simulink model "TriTiltPro_V3"  (R2019a)
settings: Solver=ode15s  StartTime=0.0  StopTime=1  RelTol=1e-3  EnableMultiTasking=on
undefined symbols (not defined in the file or in its folder): magnitude, sigbuilder_block, X, Y, Z
libraries: sm_lib x405, nesl_utility x28, simulink x13, fl_lib x7, fl_ps_legacy_lib x6, sharedtransform x1, Multibody_Multiphysics_Lib x1
(part 1 of 9)
settings Model: Creator=Administrator  LastModifiedBy=SomefunAgba
settings SolverCC: InitialStep=0.001  ZeroCrossControl=EnableAll  ZeroCrossAlgorithm=Adaptive  InsertRTBMode=Never (minimum delay)
settings DataIOCC: LimitDataPoints=on  SaveFinalState=on  SaveFormat=StructureWithTime  SaveState=on  SignalLogging=off  InspectSignalLogs=on  OutputOption=SpecifiedOutputTimes  OutputTimes=[0:1/30:1]
settings OptimizationCC: BlockReduction=off  BufferReuse=off  LifeSpan=1  MaxStackSize=64
settings DebuggingCC: SFUnexpectedBacktrackingDiag=warning  SFNoUnconditionalDefaultTransitionDiag=warning  ArithmeticOperatorsInVariantConditions=warning
settings HardwareCC: ProdBitPerPointer=32  ProdBitPerSizeT=32  ProdBitPerPtrDiffT=32  ProdLargestAtomicFloat=None  ProdIntDivRoundTo=Undefined  ProdEndianess=Unspecified  ProdWordSize=32  ProdHWDeviceType=Generic->Unspecified (assume 32-bit Generic)  TargetHWDeviceType=32-bit Generic
settings ModelReferenceCC: PropagateSignalLabelsOutOfModel=off
settings SFSimCC: SimUseLocalCustomCode=off  MATLABDynamicMemAlloc=off
settings RTWCC: SystemTargetFile=ert.tlc  HardwareBoard=Robot Operating System (ROS)  TLCOptions=-aInlineSetEventsForThisBaseRateFcn=TLC_FALSE -aSuppressMultiTaskScheduler=TLC_FALSE -aRateBasedStepFcn=0  TemplateMakefile=ert_default_tmf  GenerateReport=on  RTWUseLocalCustomCode=off  Toolchain=Catkin  IncludeHyperlinkInReport=on  LaunchReport=on  TargetLang=C++  GenerateTraceInfo=on  GenerateTraceReport=on  GenerateTraceReportSl=on  GenerateTraceReportSf=on  GenerateTraceReportEml=on
settings CodeAppCC: ForceParamTrailComments=on  IgnoreCustomStorageClasses=off  OperatorAnnotations=on  SimulinkDataObjDesc=on  SFDataObjDesc=on  MATLABFcnDesc=on  InsertBlockDesc=on  StateflowObjectComments=on  MATLABSourceComments=on
settings ERTTargetCC: MultiwordLength=2048
settings ConfigComp: CovMetricSettings=dw  CovHtmlReporting=on  CovSaveCumulativeToWorkspaceVar=on  CovSaveSingleToWorkspaceVar=on  CovExternalEMLEnable=off
settings SimscapeCC: SimscapeNormalizeSystem=off  SimscapeLogType=all  SimscapeLogSimulationStatistics=on  SimscapeLogOpenViewer=on
settings SimMechanicsCC: VisDuringSimulation=on
settings ConfigurationSet: Description=SimMechanics 2G
settings ExplorerConfigSet: InternalSimMechanicsExplorerSettings="<ExplorerConfiguration><canonicalview>planar_xy</canonicalview><AnimationSetting><BasePlaybackSpeed>1.0</BasePlaybackSpeed><PlaybackSpeedFactor>1.0</PlaybackSpeedFactor></AnimationSetting><TilePanel><TileInfo><Tiles Columns=\"1\" Count=\"1\" Rows=\"1\"><Column Left=\"2\" Weight=\"1\"/><Column Left=\"705\"/><Row Top=\"2\" Weight=\"1\"/><Row Top=\"457\"/><Tile Height=\"1\" Width=\"1\" X=\"0\" Y=\"0\"/></Tiles></TileInfo><SceneInfo><SceneViewer><BGColor><R>0.60000002384185791</R><G>0.80000001192092896</G><B>1</B></BGColor><Camera><Position><X>369622.51927765959</X><Y>14452.522627350738</Y><Z>-4093.5800779968113</Z></Position><Center><X>-0.26213935017585754</X><Y>0.48995256423950195</Y><Z>-0.58916831016540527</Z></Center><Up><X>-0.039071238740294556</X><Y>0.99923641605206415</Y><Z>-0.00015211418458100246</Z></Up><Left>-1.18166543841362</Left><Right>1.18166543841362</Right><Bottom>-0.63869556784629822</Bottom><Top>0.63869556784629822</Top></Camera></SceneViewer></SceneInfo></TilePanel></ExplorerConfiguration>"

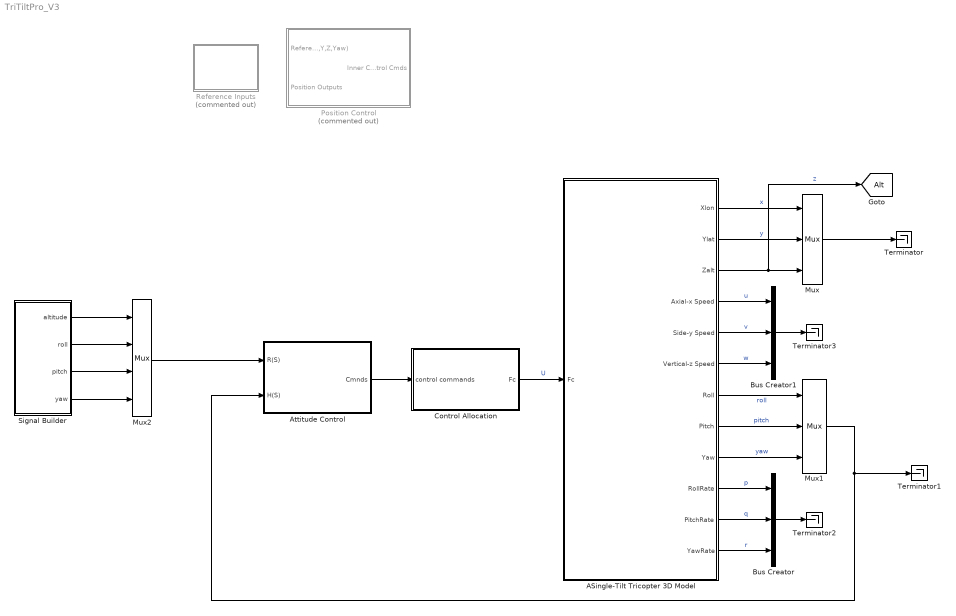
== system TriTiltPro_V3 ==
  ASingle-Tilt Tricopter 3D Model : Subsystem
  Attitude Control : Subsystem
  Bus Creator : BusCreator  Inputs=3
  Bus Creator1 : BusCreator  Inputs=3
  Control Allocation : Subsystem
  Mux : Mux  Inputs=3
  Mux1 : Mux  Inputs=3
  Mux2 : Mux
  Position Control : Subsystem  Commented=on
  Reference Inputs : Subsystem  Commented=on
  Signal Builder : Subsystem  Tag=STV Subsys  LoadFcn=sigbuilder_block('load');  StartFcn=sigbuilder_block('start');  StopFcn=sigbuilder_block('stop');  ClipboardFcn=sigbuilder_block('clipboard');  mask(Sigbuilder block){tuvar=[0:10]}
      mask help: Simulink:masks:SigbuilderBlock_MD
      mask init:
      | if ~strcmp(get_param(bdroot(gcbh),'SimulationStatus'),'stopped') tuvar = sigbuilder_block('maskInit'); end
      settings: CopyFcn=sigbuilder_block('copy');  DeleteFcn=sigbuilder_block('delete');  ModelCloseFcn=sigbuilder_block('modelClose');  PreSaveFcn=sigbuilder_block('preSave');  PauseFcn=sigbuilder_block('pause');  ContinueFcn=sigbuilder_block('continue');  NameChangeFcn=sigbuilder_block('namechange');  OpenFcn=sigbuilder_block('open',[299.25 91.5 558 358.5 ]);  CloseFcn=sigbuilder_block('close');
      mask Display: plot(0, 0, 100, 100,[2, 2, 32, 32, 2], [68, 8, 8, 68, 68],[32, 2], [38, 38], [32, 19, 2],[53, 60, 44], [32, 17, 17, 2],[16, 16, 31, 31]);txt = getActiveGroup(gcbh);text(2, 100, txt,'verticalAlignment', 'top');
  Terminator{,1..3} (4 alike) : Terminator
  tag scope: Alt=global
  wires:
  ASingle-Tilt Tricopter 3D Model/12(YawRate) -> Bus Creator/3  "r"
  ASingle-Tilt Tricopter 3D Model/11(PitchRate) -> Bus Creator/2  "q"
  ASingle-Tilt Tricopter 3D Model/10(RollRate) -> Bus Creator/1  "p"
  ASingle-Tilt Tricopter 3D Model/9(Yaw) -> Mux1/3  "yaw"
  ASingle-Tilt Tricopter 3D Model/8(Pitch) -> Mux1/2  "pitch"
  ASingle-Tilt Tricopter 3D Model/7(Roll) -> Mux1/1  "roll"
  ASingle-Tilt Tricopter 3D Model/6(Vertical-z Speed) -> Bus Creator1/3  "w"
  ASingle-Tilt Tricopter 3D Model/5(Side-y Speed) -> Bus Creator1/2  "v"
  ASingle-Tilt Tricopter 3D Model/4(Axial-x Speed) -> Bus Creator1/1  "u"
  ASingle-Tilt Tricopter 3D Model/3(Zalt) -> [Alt], Mux/3  "z"
  ASingle-Tilt Tricopter 3D Model/2(Ylat) -> Mux/2  "y"
  ASingle-Tilt Tricopter 3D Model/1(Xlon) -> Mux/1  "x"
  Mux/1 -> Terminator/1
  Mux1/1 -> Attitude Control/2(H(S)), Terminator1/1
  Control Allocation/1(Fc) -> ASingle-Tilt Tricopter 3D Model/1(Fc)  "U"
  Attitude Control/1(Cmnds) -> Control Allocation/1(control commands)
  Mux2/1 -> Attitude Control/1(R(S))
  Signal Builder/1(altitude) -> Mux2/1
  Signal Builder/2(roll) -> Mux2/2
  Signal Builder/3(pitch) -> Mux2/3
  Signal Builder/4(yaw) -> Mux2/4
  Bus Creator/1 -> Terminator2/1
  Bus Creator1/1 -> Terminator3/1

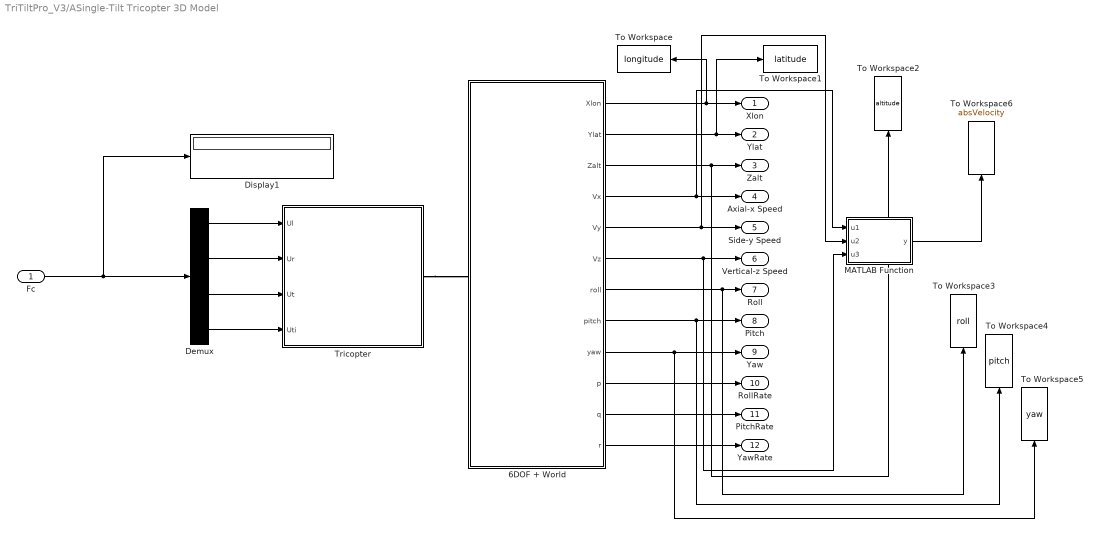
== system TriTiltPro_V3/ASingle-Tilt Tricopter 3D Model ==
  Fc : Inport
  6DOF + World : Subsystem
  Demux : Demux
  Display1 : Display
  MATLAB Function : MATLAB Function  TreatAsAtomicUnit=on
  To Workspace : ToWorkspace  VariableName=longitude  SampleTime=-1
  To Workspace1 : ToWorkspace  VariableName=latitude  SampleTime=-1
  To Workspace2 : ToWorkspace  VariableName=altitude  SampleTime=-1
  To Workspace3 : ToWorkspace  VariableName=roll  SampleTime=-1
  To Workspace4 : ToWorkspace  VariableName=pitch  SampleTime=-1
  To Workspace5 : ToWorkspace  VariableName=yaw  SampleTime=-1
  To Workspace6 : ToWorkspace  VariableName=absVelocity  SampleTime=-1
  Tricopter : Subsystem
  Xlon : Outport
  Ylat : Outport  Port=2
  Zalt : Outport  Port=3
  Axial-x Speed : Outport  Port=4
  Side-y Speed : Outport  Port=5
  Vertical-z Speed : Outport  Port=6
  Roll : Outport  Port=7
  Pitch : Outport  Port=8
  Yaw : Outport  Port=9
  RollRate : Outport  Port=10
  PitchRate : Outport  Port=11
  YawRate : Outport  Port=12
  wires:
  6DOF + World/9(yaw) -> To Workspace5/1, Yaw/1
  6DOF + World/10(p) -> RollRate/1
  6DOF + World/4(Vx) -> MATLAB Function/1(u1), Axial-x Speed/1
  6DOF + World/3(Zalt) -> To Workspace2/1, Zalt/1
  6DOF + World/11(q) -> PitchRate/1
  6DOF + World/12(r) -> YawRate/1
  6DOF + World/6(Vz) -> MATLAB Function/3(u3), Vertical-z Speed/1
  6DOF + World/2(Ylat) -> To Workspace1/1, Ylat/1
  6DOF + World/7(roll) -> To Workspace3/1, Roll/1
  6DOF + World/8(pitch) -> To Workspace4/1, Pitch/1
  6DOF + World/5(Vy) -> MATLAB Function/2(u2), Side-y Speed/1
  6DOF + World/1(Xlon) -> To Workspace/1, Xlon/1
  Demux/3 -> Tricopter/3(Ut)
  Demux/1 -> Tricopter/1(Ul)
  Demux/4 -> Tricopter/4(Uti)
  Demux/2 -> Tricopter/2(Ur)
  Fc/1 -> Display1/1, Demux/1
  MATLAB Function/1(y) -> To Workspace6/1
  connections:
  Tricopter/RConn1 -- 6DOF + World/LConn1

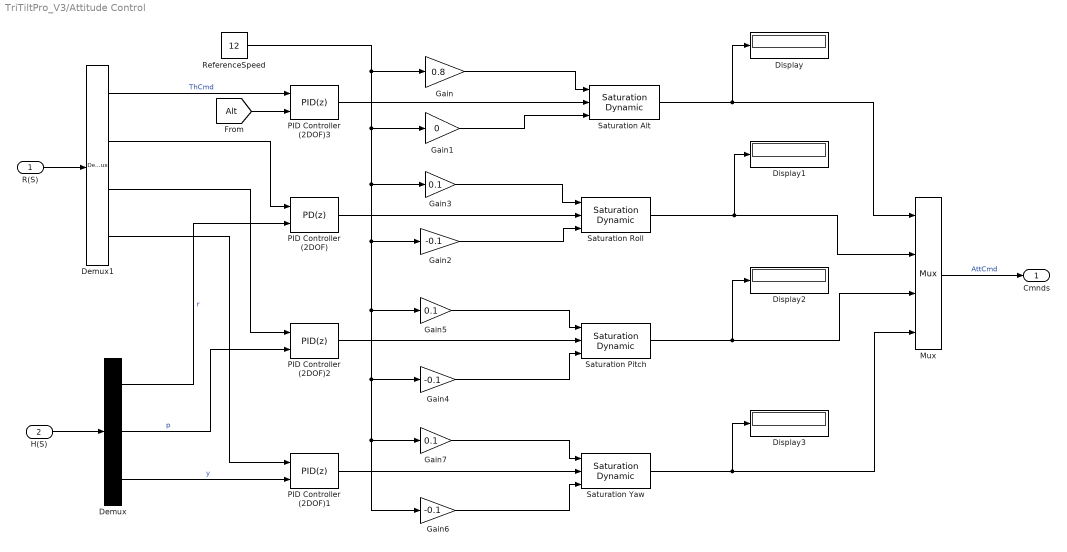
== system TriTiltPro_V3/Attitude Control ==
  R(S) : Inport
  H(S) : Inport  Port=2
  Demux : Demux  Outputs=3
  Demux1 : Demux
  Display{,1..3} (4 alike) : Display
  Gain : Gain  Gain=0.8
  Gain1 : Gain  Gain=0
  Gain2 : Gain  Gain=-0.1
  Gain3 : Gain  Gain=0.1
  Gain4 : Gain  Gain=-0.1
  Gain5 : Gain  Gain=0.1
  Gain6 : Gain  Gain=-0.1
  Gain7 : Gain  Gain=0.1
  Mux : Mux
  PID Controller (2DOF) : simulink/Continuous/PID Controller (2DOF)  Controller=PD  Form=Parallel  TimeDomain=Discrete-time  SampleTime=0.001  IntegratorMethod=Forward Euler  FilterMethod=Forward Euler  ControllerParametersSource=internal  P=21.0891711051547  I=1  D=0  UseFilter=on  N=100  b=0  c=1  TunerSelectOption=Transfer Function Based (PID Tuner App)  InitialConditionSource=internal  InitialConditionForIntegrator=0  InitialConditionForFilter=0  DifferentiatorICPrevScaledInput=0  ExternalReset=none  TrackingMode=off  Kt=1  LimitOutput=off  UpperSaturationLimit=inf  LowerSaturationLimit=-inf  LinearizeAsGain=on  AntiWindupMode=none  Kb=1  POutMin=[]  POutMax=[]  IOutMin=[]  IOutMax=[]  DOutMin=[]  DOutMax=[]  NOutMin=[]  NOutMax=[]  bOutMin=[]  bOutMax=[]  cOutMin=[]  cOutMax=[]  SumOutMin=[]  SumOutMax=[]  SaturationOutMin=[]  SaturationOutMax=[]  PParamMin=[]  PParamMax=[]  IParamMin=[]  IParamMax=[]  DParamMin=[]  DParamMax=[]  NParamMin=[]  NParamMax=[]  bParamMin=[]  bParamMax=[]  cParamMin=[]  cParamMax=[]  KbParamMin=[]  KbParamMax=[]  KtParamMin=[]  KtParamMax=[]  KbOutMin=[]  KbOutMax=[]  KtOutMin=[]  KtOutMax=[]  IntegratorOutMin=[]  IntegratorOutMax=[]  FilterOutMin=[]  FilterOutMax=[]  SumI1OutMin=[]  SumI1OutMax=[]  SumI2OutMin=[]  SumI2OutMax=[]  SumI3OutMin=[]  SumI3OutMax=[]  SumI4OutMin=[]  SumI4OutMax=[]  SumDOutMin=[]  SumDOutMax=[]  Sum1OutMin=[]  Sum1OutMax=[]  Sum2OutMin=[]  Sum2OutMax=[]  Sum3OutMin=[]  Sum3OutMax=[]  DifferentiatorOutMin=[]  DifferentiatorOutMax=[]  FilterDiffOutCoefMin=[]  FilterDiffOutCoefMax=[]  ReciprocalOutMin=[]  ReciprocalOutMax=[]  SumDenOutMin=[]  SumDenOutMax=[]  SumNumOutMin=[]  SumNumOutMax=[]  DivideOutMin=[]  DivideOutMax=[]  IntegratorContinuousStateAttributes=''  IntegratorStateMustResolveToSignalObject=off  IntegratorRTWStateStorageClass=Auto  FilterContinuousStateAttributes=''  FilterStateMustResolveToSignalObject=off  FilterRTWStateStorageClass=Auto  ParallelPVariant=InternalParameters  IdealPVariant=Disabled  IVariant=Disabled  DVariant=InternalParameters  bVariant=InternalParameters  cVariant=InternalParameters  IntegratorVariant=Disabled  SatVariant=Disabled  AWVariant=Disabled  PCopyVariant=Disabled  TRVariant=Disabled  FdbkBlocksVariant=Forward  IdealPFdbkVariant=Disabled  SatFdbkVariant=Disabled  DerivativeFilterVariant=ForwardEulerFilter  NVariant=InternalParameters  NCopyVariant=Disabled  FilterICVariant=InternalICsFilter  IntegratorICVariant=Disabled  ExternalResetVariant=Disabled  TRSumVariant=Passthrough  SumFdbkVariant=Disabled  SumVariant=Sum_PD
  PID Controller (2DOF)1 : simulink/Continuous/PID Controller (2DOF)  Controller=PID  Form=Parallel  TimeDomain=Discrete-time  SampleTime=0.001  IntegratorMethod=Forward Euler  FilterMethod=Forward Euler  ControllerParametersSource=internal  P=0.02  I=0.4  D=0.001  UseFilter=on  N=1730.43460231117  b=0.949409560304364  c=0.478998391491009  TunerSelectOption=Transfer Function Based (PID Tuner App)  InitialConditionSource=internal  InitialConditionForIntegrator=0  InitialConditionForFilter=0  DifferentiatorICPrevScaledInput=0  ExternalReset=none  TrackingMode=off  Kt=1  LimitOutput=off  UpperSaturationLimit=inf  LowerSaturationLimit=-inf  LinearizeAsGain=on  AntiWindupMode=none  Kb=1  POutMin=[]  POutMax=[]  IOutMin=[]  IOutMax=[]  DOutMin=[]  DOutMax=[]  NOutMin=[]  NOutMax=[]  bOutMin=[]  bOutMax=[]  cOutMin=[]  cOutMax=[]  SumOutMin=[]  SumOutMax=[]  SaturationOutMin=[]  SaturationOutMax=[]  PParamMin=[]  PParamMax=[]  IParamMin=[]  IParamMax=[]  DParamMin=[]  DParamMax=[]  NParamMin=[]  NParamMax=[]  bParamMin=[]  bParamMax=[]  cParamMin=[]  cParamMax=[]  KbParamMin=[]  KbParamMax=[]  KtParamMin=[]  KtParamMax=[]  KbOutMin=[]  KbOutMax=[]  KtOutMin=[]  KtOutMax=[]  IntegratorOutMin=[]  IntegratorOutMax=[]  FilterOutMin=[]  FilterOutMax=[]  SumI1OutMin=[]  SumI1OutMax=[]  SumI2OutMin=[]  SumI2OutMax=[]  SumI3OutMin=[]  SumI3OutMax=[]  SumI4OutMin=[]  SumI4OutMax=[]  SumDOutMin=[]  SumDOutMax=[]  Sum1OutMin=[]  Sum1OutMax=[]  Sum2OutMin=[]  Sum2OutMax=[]  Sum3OutMin=[]  Sum3OutMax=[]  DifferentiatorOutMin=[]  DifferentiatorOutMax=[]  FilterDiffOutCoefMin=[]  FilterDiffOutCoefMax=[]  ReciprocalOutMin=[]  ReciprocalOutMax=[]  SumDenOutMin=[]  SumDenOutMax=[]  SumNumOutMin=[]  SumNumOutMax=[]  DivideOutMin=[]  DivideOutMax=[]  IntegratorContinuousStateAttributes=''  IntegratorStateMustResolveToSignalObject=off  IntegratorRTWStateStorageClass=Auto  FilterContinuousStateAttributes=''  FilterStateMustResolveToSignalObject=off  FilterRTWStateStorageClass=Auto  ParallelPVariant=InternalParameters  IdealPVariant=Disabled  IVariant=InternalParameters  DVariant=InternalParameters  bVariant=InternalParameters  cVariant=InternalParameters  IntegratorVariant=Discrete  SatVariant=Disabled  AWVariant=Passthrough  PCopyVariant=Disabled  TRVariant=Disabled  FdbkBlocksVariant=Forward  IdealPFdbkVariant=Disabled  SatFdbkVariant=Disabled  DerivativeFilterVariant=ForwardEulerFilter  NVariant=InternalParameters  NCopyVariant=Disabled  FilterICVariant=InternalICsFilter  IntegratorICVariant=InternalICs  ExternalResetVariant=Disabled  TRSumVariant=Passthrough  SumFdbkVariant=Disabled  SumVariant=Sum_PID
  PID Controller (2DOF)2 : simulink/Continuous/PID Controller (2DOF)  Controller=PID  Form=Parallel  TimeDomain=Discrete-time  SampleTime=0.001  IntegratorMethod=Forward Euler  FilterMethod=Forward Euler  ControllerParametersSource=internal  P=0.02  I=0.4  D=0.001  UseFilter=on  N=100  b=1  c=1  TunerSelectOption=Transfer Function Based (PID Tuner App)  InitialConditionSource=internal  InitialConditionForIntegrator=0  InitialConditionForFilter=0  DifferentiatorICPrevScaledInput=0  ExternalReset=none  TrackingMode=off  Kt=1  LimitOutput=off  UpperSaturationLimit=inf  LowerSaturationLimit=-inf  LinearizeAsGain=on  AntiWindupMode=none  Kb=1  POutMin=[]  POutMax=[]  IOutMin=[]  IOutMax=[]  DOutMin=[]  DOutMax=[]  NOutMin=[]  NOutMax=[]  bOutMin=[]  bOutMax=[]  cOutMin=[]  cOutMax=[]  SumOutMin=[]  SumOutMax=[]  SaturationOutMin=[]  SaturationOutMax=[]  PParamMin=[]  PParamMax=[]  IParamMin=[]  IParamMax=[]  DParamMin=[]  DParamMax=[]  NParamMin=[]  NParamMax=[]  bParamMin=[]  bParamMax=[]  cParamMin=[]  cParamMax=[]  KbParamMin=[]  KbParamMax=[]  KtParamMin=[]  KtParamMax=[]  KbOutMin=[]  KbOutMax=[]  KtOutMin=[]  KtOutMax=[]  IntegratorOutMin=[]  IntegratorOutMax=[]  FilterOutMin=[]  FilterOutMax=[]  SumI1OutMin=[]  SumI1OutMax=[]  SumI2OutMin=[]  SumI2OutMax=[]  SumI3OutMin=[]  SumI3OutMax=[]  SumI4OutMin=[]  SumI4OutMax=[]  SumDOutMin=[]  SumDOutMax=[]  Sum1OutMin=[]  Sum1OutMax=[]  Sum2OutMin=[]  Sum2OutMax=[]  Sum3OutMin=[]  Sum3OutMax=[]  DifferentiatorOutMin=[]  DifferentiatorOutMax=[]  FilterDiffOutCoefMin=[]  FilterDiffOutCoefMax=[]  ReciprocalOutMin=[]  ReciprocalOutMax=[]  SumDenOutMin=[]  SumDenOutMax=[]  SumNumOutMin=[]  SumNumOutMax=[]  DivideOutMin=[]  DivideOutMax=[]  IntegratorContinuousStateAttributes=''  IntegratorStateMustResolveToSignalObject=off  IntegratorRTWStateStorageClass=Auto  FilterContinuousStateAttributes=''  FilterStateMustResolveToSignalObject=off  FilterRTWStateStorageClass=Auto  ParallelPVariant=InternalParameters  IdealPVariant=Disabled  IVariant=InternalParameters  DVariant=InternalParameters  bVariant=InternalParameters  cVariant=InternalParameters  IntegratorVariant=Discrete  SatVariant=Disabled  AWVariant=Passthrough  PCopyVariant=Disabled  TRVariant=Disabled  FdbkBlocksVariant=Forward  IdealPFdbkVariant=Disabled  SatFdbkVariant=Disabled  DerivativeFilterVariant=ForwardEulerFilter  NVariant=InternalParameters  NCopyVariant=Disabled  FilterICVariant=InternalICsFilter  IntegratorICVariant=InternalICs  ExternalResetVariant=Disabled  TRSumVariant=Passthrough  SumFdbkVariant=Disabled  SumVariant=Sum_PID
  PID Controller (2DOF)3 : simulink/Continuous/PID Controller (2DOF)  Controller=PID  Form=Parallel  TimeDomain=Discrete-time  SampleTime=0.001  IntegratorMethod=Forward Euler  FilterMethod=Forward Euler  ControllerParametersSource=internal  P=15.9810269634034  I=1121.61470890408  D=0  UseFilter=on  N=100  b=1  c=1  TunerSelectOption=Transfer Function Based (PID Tuner App)  InitialConditionSource=internal  InitialConditionForIntegrator=0  InitialConditionForFilter=0  DifferentiatorICPrevScaledInput=0  ExternalReset=none  TrackingMode=off  Kt=1  LimitOutput=off  UpperSaturationLimit=inf  LowerSaturationLimit=-inf  LinearizeAsGain=on  AntiWindupMode=none  Kb=1  POutMin=[]  POutMax=[]  IOutMin=[]  IOutMax=[]  DOutMin=[]  DOutMax=[]  NOutMin=[]  NOutMax=[]  bOutMin=[]  bOutMax=[]  cOutMin=[]  cOutMax=[]  SumOutMin=[]  SumOutMax=[]  SaturationOutMin=[]  SaturationOutMax=[]  PParamMin=[]  PParamMax=[]  IParamMin=[]  IParamMax=[]  DParamMin=[]  DParamMax=[]  NParamMin=[]  NParamMax=[]  bParamMin=[]  bParamMax=[]  cParamMin=[]  cParamMax=[]  KbParamMin=[]  KbParamMax=[]  KtParamMin=[]  KtParamMax=[]  KbOutMin=[]  KbOutMax=[]  KtOutMin=[]  KtOutMax=[]  IntegratorOutMin=[]  IntegratorOutMax=[]  FilterOutMin=[]  FilterOutMax=[]  SumI1OutMin=[]  SumI1OutMax=[]  SumI2OutMin=[]  SumI2OutMax=[]  SumI3OutMin=[]  SumI3OutMax=[]  SumI4OutMin=[]  SumI4OutMax=[]  SumDOutMin=[]  SumDOutMax=[]  Sum1OutMin=[]  Sum1OutMax=[]  Sum2OutMin=[]  Sum2OutMax=[]  Sum3OutMin=[]  Sum3OutMax=[]  DifferentiatorOutMin=[]  DifferentiatorOutMax=[]  FilterDiffOutCoefMin=[]  FilterDiffOutCoefMax=[]  ReciprocalOutMin=[]  ReciprocalOutMax=[]  SumDenOutMin=[]  SumDenOutMax=[]  SumNumOutMin=[]  SumNumOutMax=[]  DivideOutMin=[]  DivideOutMax=[]  IntegratorContinuousStateAttributes=''  IntegratorStateMustResolveToSignalObject=off  IntegratorRTWStateStorageClass=Auto  FilterContinuousStateAttributes=''  FilterStateMustResolveToSignalObject=off  FilterRTWStateStorageClass=Auto  ParallelPVariant=InternalParameters  IdealPVariant=Disabled  IVariant=InternalParameters  DVariant=InternalParameters  bVariant=InternalParameters  cVariant=InternalParameters  IntegratorVariant=Discrete  SatVariant=Disabled  AWVariant=Passthrough  PCopyVariant=Disabled  TRVariant=Disabled  FdbkBlocksVariant=Forward  IdealPFdbkVariant=Disabled  SatFdbkVariant=Disabled  DerivativeFilterVariant=ForwardEulerFilter  NVariant=InternalParameters  NCopyVariant=Disabled  FilterICVariant=InternalICsFilter  IntegratorICVariant=InternalICs  ExternalResetVariant=Disabled  TRSumVariant=Passthrough  SumFdbkVariant=Disabled  SumVariant=Sum_PID
  ReferenceSpeed : Constant  Value=12
  Saturation Alt : simulink/Discontinuities/Saturation Dynamic  OutMin=[]  OutMax=[]  OutDataTypeStr=Inherit: Same as second input  OutDataType=fixdt(1, 16)  OutScaling=2^-10  DoSatur=off
  Saturation Pitch : simulink/Discontinuities/Saturation Dynamic  OutMin=[]  OutMax=[]  OutDataTypeStr=Inherit: Same as second input  OutDataType=fixdt(1, 16)  OutScaling=2^-10  DoSatur=off
  Saturation Roll : simulink/Discontinuities/Saturation Dynamic  OutMin=[]  OutMax=[]  OutDataTypeStr=Inherit: Same as second input  OutDataType=fixdt(1, 16)  OutScaling=2^-10  DoSatur=off
  Saturation Yaw : simulink/Discontinuities/Saturation Dynamic  OutMin=[]  OutMax=[]  OutDataTypeStr=Inherit: Same as second input  OutDataType=fixdt(1, 16)  OutScaling=2^-10  DoSatur=off
  Cmnds : Outport
  wires:
  H(S)/1 -> Demux/1
  R(S)/1 -> Demux1/1
  Gain/1 -> Saturation Alt/1
  Gain1/1 -> Saturation Alt/3
  PID Controller (2DOF)3/1 -> Saturation Alt/2
  PID Controller (2DOF)/1 -> Saturation Roll/2
  Gain3/1 -> Saturation Roll/1
  Gain2/1 -> Saturation Roll/3
  PID Controller (2DOF)2/1 -> Saturation Pitch/2
  Gain5/1 -> Saturation Pitch/1
  Gain4/1 -> Saturation Pitch/3
  Mux/1 -> Cmnds/1  "AttCmd"
  Saturation Alt/1 -> Display/1, Mux/1
  Saturation Roll/1 -> Mux/2, Display1/1
  Saturation Pitch/1 -> Mux/3, Display2/1
  ReferenceSpeed/1 -> Gain7/1, Gain6/1, Gain4/1, Gain5/1, Gain2/1, Gain3/1, Gain1/1, Gain/1
  PID Controller (2DOF)1/1 -> Saturation Yaw/2
  Gain7/1 -> Saturation Yaw/1
  Gain6/1 -> Saturation Yaw/3
  Saturation Yaw/1 -> Mux/4, Display3/1
  Demux1/1 -> PID Controller (2DOF)3/1  "ThCmd"
  Demux/3 -> PID Controller (2DOF)1/2  "y"
  Demux1/4 -> PID Controller (2DOF)1/1
  Demux/2 -> PID Controller (2DOF)2/2  "p"
  Demux1/3 -> PID Controller (2DOF)2/1
  Demux/1 -> PID Controller (2DOF)/2  "r"
  Demux1/2 -> PID Controller (2DOF)/1
  [Alt] -> PID Controller (2DOF)3/2

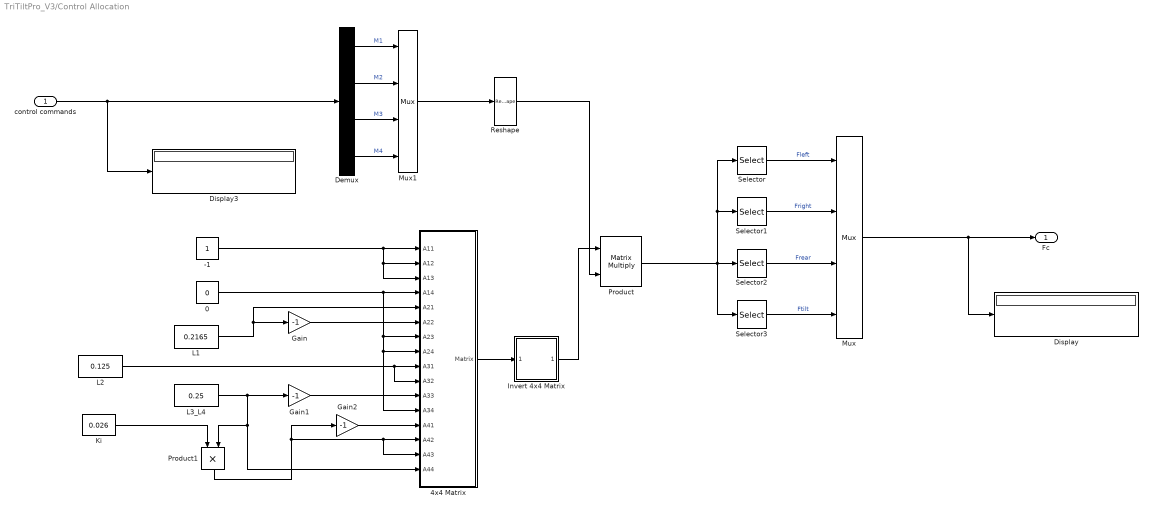
== system TriTiltPro_V3/Control Allocation ==
  control commands : Inport
  -1 : Constant
  0 : Constant  Value=0
  4x4 Matrix : Subsystem
      mask Display:
      | port_label('input',1,'A_{11}','texmode','on');
      | port_label('input',2,'A_{12}','texmode','on');
      | port_label('input',3,'A_{13}','texmode','on');
      | port_label('input',4,'A_{14}','texmode','on');
      | port_label('input',5,'A_{21}','texmode','on');
      | port_label('input',6,'A_{22}','texmode','on');
      | port_label('input',7,'A_{23}','texmode','on');
      | port_label('input',8,'A_{24}','texmode','on');
      | port_label('input',9,'A_{31}','texmode','on');
      | port_label('input',10,'A_{32}','texmode','on');
      | port_label('input',11,'A_{33}','texmode','on');
      | port_label('input',12,'A_{34}','texmode','on');
      | port_label('input',13,'A_{41}','texmode','on');
      | port_label('input',14,'A_{42}','texmode','on');
      | port_label('input',15,'A_{43}','texmode','on');
      | port_label('input',16,'A_{44}','texmode','on');
      | port_label('output',1,'A','texmode','on');
  Demux : Demux
  Display : Display
  Display3 : Display
  Gain : Gain  Gain=-1
  Gain1 : Gain  Gain=-1
  Gain2 : Gain  Gain=-1
  Invert 4x4 Matrix : Subsystem
      mask Display: fprintf('inv(A)\n(4x4)');
  Ki : Constant  Value=0.026
  L1 : Constant  Value=0.2165
  L2 : Constant  Value=0.125
  L3_L4 : Constant  Value=0.25
  Mux : Mux
  Mux1 : Mux
  Product : Product  Inputs=**  Multiplication=Matrix(*)
  Product1 : Product
  Reshape : Reshape  OutputDimensionality=Customize  OutputDimensions=[4,1]
  Selector : Selector  InputPortWidth=4  IndexOptions=Index vector (dialog)  Indices=[1]  OutputSizes=1
  Selector1 : Selector  InputPortWidth=4  IndexOptions=Index vector (dialog)  Indices=[2]  OutputSizes=1
  Selector2 : Selector  InputPortWidth=4  IndexOptions=Index vector (dialog)  Indices=[3]  OutputSizes=1
  Selector3 : Selector  InputPortWidth=4  IndexOptions=Index vector (dialog)  Indices=[4]  OutputSizes=1
  Fc : Outport
  wires:
  -1/1 -> 4x4 Matrix/3(A13), 4x4 Matrix/2(A12), 4x4 Matrix/1(A11)
  Product/1 -> Selector/1, Selector1/1, Selector3/1, Selector2/1
  Selector/1 -> Mux/1  "Fleft"
  Selector1/1 -> Mux/2  "Fright"
  Selector2/1 -> Mux/3  "Frear"
  Selector3/1 -> Mux/4  "Ftilt"
  L1/1 -> 4x4 Matrix/5(A21), Gain/1
  0/1 -> 4x4 Matrix/8(A24), 4x4 Matrix/12(A34), 4x4 Matrix/7(A23), 4x4 Matrix/4(A14)
  Reshape/1 -> Product/2
  Invert 4x4 Matrix/1(InvMatrix) -> Product/1
  4x4 Matrix/1(Matrix) -> Invert 4x4 Matrix/1(MatrixIn)
  Demux/1 -> Mux1/1  "M1"
  Demux/2 -> Mux1/2  "M2"
  Demux/3 -> Mux1/3  "M3"
  Demux/4 -> Mux1/4  "M4"
  Mux1/1 -> Reshape/1
  Mux/1 -> Display/1, Fc/1
  control commands/1 -> Display3/1, Demux/1
  L2/1 -> 4x4 Matrix/10(A32), 4x4 Matrix/9(A31)
  L3_L4/1 -> Product1/2, 4x4 Matrix/16(A44), Gain1/1
  Ki/1 -> Product1/1
  Gain/1 -> 4x4 Matrix/6(A22)
  Gain1/1 -> 4x4 Matrix/11(A33)
  Gain2/1 -> 4x4 Matrix/13(A41)
  Product1/1 -> Gain2/1, 4x4 Matrix/14(A42), 4x4 Matrix/15(A43)

== system TriTiltPro_V3/Position Control ==
  Reference Cmds(X,Y,Z,Yaw) : Inport
  Position Outputs : Inport  Port=2
  Demux : Demux
  Mux : Mux  Inputs=3
  Outer Error Ports : Subsystem
  PID Controller : Subsystem
  Position Control Allocation : Subsystem
  Inner Control Cmds : Outport
  wires:
  Mux/1 -> Outer Error Ports/1(Reference Inputs)
  Position Outputs/1 -> Outer Error Ports/2(Outputs)
  Demux/4 -> PID Controller/2(Yaw Ref)  "Yaw Reference"
  Outer Error Ports/1(Errors) -> PID Controller/1(Errors)
  PID Controller/1(Thrustsxyz) -> Position Control Allocation/1(ThrustsXYZ)
  PID Controller/2(YawRef) -> Position Control Allocation/2(Yaw Ref)
  Position Control Allocation/1(Desired Cmds) -> Inner Control Cmds/1
  Demux/3 -> Mux/3
  Demux/1 -> Mux/1
  Demux/2 -> Mux/2
  Reference Cmds(X,Y,Z,Yaw)/1 -> Demux/1

== system TriTiltPro_V3/Reference Inputs ==
  Inputs1 : Subsystem  Commented=on
  Signal Builder : Subsystem  Tag=STV Subsys  Commented=on  LoadFcn=sigbuilder_block('load');  StartFcn=sigbuilder_block('start');  StopFcn=sigbuilder_block('stop');  ClipboardFcn=sigbuilder_block('clipboard');  mask(Sigbuilder block){tuvar=[0:10]}
      mask help: Simulink:masks:SigbuilderBlock_MD
      mask init:
      | if ~strcmp(get_param(bdroot(gcbh),'SimulationStatus'),'stopped') tuvar = sigbuilder_block('maskInit'); end
      settings: CopyFcn=sigbuilder_block('copy');  DeleteFcn=sigbuilder_block('delete');  ModelCloseFcn=sigbuilder_block('modelClose');  PreSaveFcn=sigbuilder_block('preSave');  PauseFcn=sigbuilder_block('pause');  ContinueFcn=sigbuilder_block('continue');  NameChangeFcn=sigbuilder_block('namechange');  OpenFcn=sigbuilder_block('open',[437.6 199.2 550.4 400 ]);  CloseFcn=sigbuilder_block('close');
      mask Display: plot(0, 0, 100, 100,[2, 2, 32, 32, 2], [68, 8, 8, 68, 68],[32, 2], [38, 38], [32, 19, 2],[53, 60, 44], [32, 17, 17, 2],[16, 16, 31, 31]);txt = getActiveGroup(gcbh);text(2, 100, txt,'verticalAlignment', 'top');
  Signal Builder1 : Subsystem  Tag=STV Subsys  Commented=on  LoadFcn=sigbuilder_block('load');  StartFcn=sigbuilder_block('start');  StopFcn=sigbuilder_block('stop');  ClipboardFcn=sigbuilder_block('clipboard');  mask(Sigbuilder block){tuvar=[0:10]}
      mask help: Simulink:masks:SigbuilderBlock_MD
      mask init:
      | if ~strcmp(get_param(bdroot(gcbh),'SimulationStatus'),'stopped') tuvar = sigbuilder_block('maskInit'); end
      settings: CopyFcn=sigbuilder_block('copy');  DeleteFcn=sigbuilder_block('delete');  ModelCloseFcn=sigbuilder_block('modelClose');  PreSaveFcn=sigbuilder_block('preSave');  PauseFcn=sigbuilder_block('pause');  ContinueFcn=sigbuilder_block('continue');  NameChangeFcn=sigbuilder_block('namechange');  OpenFcn=sigbuilder_block('open',[437.6 199.2 550.4 400 ]);  CloseFcn=sigbuilder_block('close');
      mask Display: plot(0, 0, 100, 100,[2, 2, 32, 32, 2], [68, 8, 8, 68, 68],[32, 2], [38, 38], [32, 19, 2],[53, 60, 44], [32, 17, 17, 2],[16, 16, 31, 31]);txt = getActiveGroup(gcbh);text(2, 100, txt,'verticalAlignment', 'top');

== system TriTiltPro_V3/Signal Builder ==
  Demux : Demux  Tag=STV Demux
  FromWs : FromWorkspace  Tag=STV FromWs  VariableName=tuvar  SampleTime=0
      SigBuilderData=|
      | common.afterFinalStr = 'Extrapolate'
      | common.sampleTime = 0
      | dataSet.timeRange = [0 2]
      | dataSet.name = 'Group 1'
      | sbobj.Groups.Name = 'Group 1'
      | sbobj.Groups.Signals(1).Name = 'altitude'
      | sbobj.Groups.Signals(1).XData = [0 0.2 0.2 2]
      | sbobj.Groups.Signals(1).YData = [0 0 1 1]
      | sbobj.Groups.Signals(2).Name = 'roll'
      | sbobj.Groups.Signals(2).XData = [0 2]
      | sbobj.Groups.Signals(2).YData = [0 0]
      | sbobj.Groups.Signals(3).Name = 'pitch'
      | sbobj.Groups.Signals(3).XData = [0 2]
      | sbobj.Groups.Signals(3).YData = [0 0]
      | sbobj.Groups.Signals(4).Name = 'yaw'
      | sbobj.Groups.Signals(4).XData = [0 2]
      | sbobj.Groups.Signals(4).YData = [0 0]
      | sbobj.Groups.TimeRange = [0 2]
  altitude : Outport  Tag=STV Outport
  roll : Outport  Tag=STV Outport  Port=2
  pitch : Outport  Tag=STV Outport  Port=3
  yaw : Outport  Tag=STV Outport  Port=4
  wires:
  FromWs/1 -> Demux/1
  Demux/1 -> altitude/1
  Demux/2 -> roll/1
  Demux/3 -> pitch/1
  Demux/4 -> yaw/1

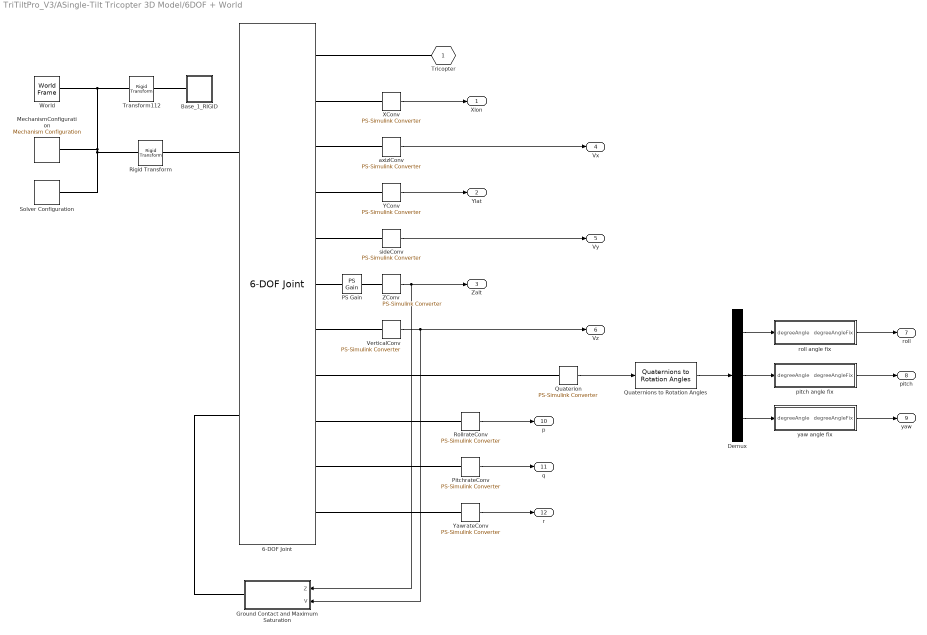
== system TriTiltPro_V3/ASingle-Tilt Tricopter 3D Model/6DOF + World ==
  6-DOF Joint : sm_lib/Joints/6-DOF Joint  SenseConstraintForce=off  SenseConstraintForceX=off  SenseConstraintForceY=off  SenseConstraintForceZ=off  SenseConstraintTorque=off  SenseConstraintTorqueX=off  SenseConstraintTorqueY=off  SenseConstraintTorqueZ=off  SenseTotalForce=off  SenseTotalForceX=off  SenseTotalForceY=off  SenseTotalForceZ=off  SenseTotalTorque=off  SenseTotalTorqueX=off  SenseTotalTorqueY=off  SenseTotalTorqueZ=off  CompositeWrenchDir=FollowerOnBase  CompositeWrenchFrame=BaseFrame  PxEquilibriumPosition=0  PxEquilibriumPositionUnits=m  PxSpringStiffness=0  PxSpringStiffnessUnits=N/m  PxDampingCoefficient=0  PxDampingCoefficientUnits=N/(m/s)  PxTorqueActuationMode=NoTorque  PxMotionActuationMode=ComputedMotion  PxSensePosition=on  PxSenseVelocity=on  PxSenseAcceleration=off  PxSenseTorqueForce=off  PxSenseLowerLimitTorqueForce=off  PxSenseUpperLimitTorqueForce=off  PxLowerLimitSpecify=off  PxLowerLimitBound=-1  PxLowerLimitBoundUnits=m  PxLowerLimitStiffness=1e6  PxLowerLimitStiffnessUnits=N/m  PxLowerLimitDamping=1e3  PxLowerLimitDampingUnits=N/(m/s)  PxLowerLimitTransitionRegionWidth=1e-4  PxLowerLimitTransitionRegionWidthUnits=m  PxUpperLimitSpecify=off  PxUpperLimitBound=1  PxUpperLimitBoundUnits=m  PxUpperLimitStiffness=1e6  PxUpperLimitStiffnessUnits=N/m  PxUpperLimitDamping=1e3  PxUpperLimitDampingUnits=N/(m/s)  PxUpperLimitTransitionRegionWidth=1e-4  PxUpperLimitTransitionRegionWidthUnits=m  PxPositionTargetSpecify=off  PxPositionTargetPriority=High  PxPositionTargetValue=0  PxPositionTargetValueUnits=m  PxVelocityTargetSpecify=off  PxVelocityTargetPriority=High  PxVelocityTargetValue=0  PxVelocityTargetValueUnits=m/s  PyEquilibriumPosition=0  PyEquilibriumPositionUnits=m  PySpringStiffness=0  PySpringStiffnessUnits=N/m  PyDampingCoefficient=0  PyDampingCoefficientUnits=N/(m/s)  PyTorqueActuationMode=NoTorque  PyMotionActuationMode=ComputedMotion  PySensePosition=on  PySenseVelocity=on  PySenseAcceleration=off  PySenseTorqueForce=off  PySenseLowerLimitTorqueForce=off  PySenseUpperLimitTorqueForce=off  PyLowerLimitSpecify=off  PyLowerLimitBound=-1  PyLowerLimitBoundUnits=m  PyLowerLimitStiffness=1e6  PyLowerLimitStiffnessUnits=N/m  PyLowerLimitDamping=1e3  PyLowerLimitDampingUnits=N/(m/s)  PyLowerLimitTransitionRegionWidth=1e-4  PyLowerLimitTransitionRegionWidthUnits=m  PyUpperLimitSpecify=off  PyUpperLimitBound=1  PyUpperLimitBoundUnits=m  PyUpperLimitStiffness=1e6  PyUpperLimitStiffnessUnits=N/m  PyUpperLimitDamping=1e3  PyUpperLimitDampingUnits=N/(m/s)  PyUpperLimitTransitionRegionWidth=1e-4  PyUpperLimitTransitionRegionWidthUnits=m  PyPositionTargetSpecify=off  PyPositionTargetPriority=High  PyPositionTargetValue=0  PyPositionTargetValueUnits=m  PyVelocityTargetSpecify=off  PyVelocityTargetPriority=High  PyVelocityTargetValue=0  PyVelocityTargetValueUnits=m/s  PzEquilibriumPosition=0  PzEquilibriumPositionUnits=m  PzSpringStiffness=0  PzSpringStiffnessUnits=N/m  PzDampingCoefficient=0  PzDampingCoefficientUnits=N/(m/s)  PzTorqueActuationMode=InputTorque  PzMotionActuationMode=ComputedMotion  PzSensePosition=on  PzSenseVelocity=on  PzSenseAcceleration=off  PzSenseTorqueForce=off  PzSenseLowerLimitTorqueForce=off  PzSenseUpperLimitTorqueForce=off  PzLowerLimitSpecify=off  PzLowerLimitBound=-1  PzLowerLimitBoundUnits=m  PzLowerLimitStiffness=1e6  PzLowerLimitStiffnessUnits=N/m  PzLowerLimitDamping=1e3  PzLowerLimitDampingUnits=N/(m/s)  PzLowerLimitTransitionRegionWidth=1e-4  PzLowerLimitTransitionRegionWidthUnits=m  PzUpperLimitSpecify=off  PzUpperLimitBound=1  PzUpperLimitBoundUnits=m  PzUpperLimitStiffness=1e6  PzUpperLimitStiffnessUnits=N/m  PzUpperLimitDamping=1e3  PzUpperLimitDampingUnits=N/(m/s)  PzUpperLimitTransitionRegionWidth=1e-4  PzUpperLimitTransitionRegionWidthUnits=m  PzPositionTargetSpecify=off  PzPositionTargetPriority=High  PzPositionTargetValue=0  PzPositionTargetValueUnits=m  PzVelocityTargetSpecify=off  PzVelocityTargetPriority=High  PzVelocityTargetValue=0  PzVelocityTargetValueUnits=m/s  SphDefPosRotationMethod=None  SphDefPosRotationAngleUnits=deg  SphDefPosRotationStandardAxis=+Z  SphDefPosRotationAngle=0.0  SphDefPosRotationArbitraryAxis=[0 0 1]  SphDefPosFollAlignAxisA=+X  SphDefPosBaseAlignAxisA=+Y  SphDefPosFollAlignAxisB=+Y  SphDefPosBaseAlignAxisB=+Z  SphDefPosRotationSequenceAxes=FollowerAxes  SphDefPosRotationSequence=XYX  SphDefPosRotationSequenceAngles=[0 0 0]  SphDefPosRotationSequenceAnglesUnits=deg  SphDefPosRotationMatrix=[1 0 0; 0 1 0; 0 0 1]  SphEqPosRotationMethod=None  SphEqPosRotationAngleUnits=deg  SphEqPosRotationStandardAxis=+Z  SphEqPosRotationAngle=0.0  SphEqPosRotationArbitraryAxis=[0 0 1]  SphEqPosFollAlignAxisA=+X  SphEqPosBaseAlignAxisA=+Y  SphEqPosFollAlignAxisB=+Y  SphEqPosBaseAlignAxisB=+Z  SphEqPosRotationSequenceAxes=FollowerAxes  SphEqPosRotationSequence=XYX  SphEqPosRotationSequenceAngles=[0 0 0]  SphEqPosRotationSequenceAnglesUnits=deg  SphEqPosRotationMatrix=[1 0 0; 0 1 0; 0 0 1]  SphSpringStiffness=0  SphSpringStiffnessUnits=N*m/deg  SphDampingCoefficient=0  SphDampingCoefficientUnits=N*m/(deg/s)  SphActuateTorqueX=off  SphActuateTorqueY=off  SphActuateTorqueZ=off  SphActuateTorque=off  SphTorqueActuationMode=NoTorque  SphMotionActuationMode=ComputedMotion  SphActuationFrame=BaseFrame  SphSensePosition=on  SphSenseVelocityX=on  SphSenseVelocityY=on  SphSenseVelocityZ=on  SphSenseVelocity=off  SphSenseAccelerationX=off  SphSenseAccelerationY=off  SphSenseAccelerationZ=off  SphSenseAcceleration=off  SphSenseTorqueX=off  SphSenseTorqueY=off  SphSenseTorqueZ=off  SphSenseTorqueForce=off  SphSenseLowerLimitTorqueMag=off  SphSenseUpperLimitTorqueMag=off  SphSensingFrame=BaseFrame  SphLowerLimitSpecify=off  SphLowerLimitBound=15  SphLowerLimitBoundUnits=deg  SphLowerLimitStiffness=1e4  SphLowerLimitStiffnessUnits=N*m/deg  SphLowerLimitDamping=10  SphLowerLimitDampingUnits=N*m/(deg/s)  SphLowerLimitTransitionRegionWidth=0.1  SphLowerLimitTransitionRegionWidthUnits=deg  SphUpperLimitSpecify=off  SphUpperLimitBound=45  SphUpperLimitBoundUnits=deg  SphUpperLimitStiffness=1e4  SphUpperLimitStiffnessUnits=N*m/deg  SphUpperLimitDamping=10  SphUpperLimitDampingUnits=N*m/(deg/s)  SphUpperLimitTransitionRegionWidth=0.1  SphUpperLimitTransitionRegionWidthUnits=deg  SphPositionTargetRotationMethod=None  SphPositionTargetRotationAngleUnits=deg  SphPositionTargetRotationStandardAxis=+Z  SphPositionTargetRotationAngle=0.0  SphPositionTargetRotationArbitraryAxis=[0 0 1]  SphPositionTargetFollAlignAxisA=+X  SphPositionTargetBaseAlignAxisA=+Y  SphPositionTargetFollAlignAxisB=+Y  SphPositionTargetBaseAlignAxisB=+Z  SphPositionTargetRotationSequenceAxes=FollowerAxes  SphPositionTargetRotationSequence=XYX  SphPositionTargetRotationSequenceAngles=[0 0 0]  SphPositionTargetRotationSequenceAnglesUnits=deg  SphPositionTargetRotationMatrix=[1 0 0; 0 1 0; 0 0 1]  SphPositionTargetSpecify=off  SphPositionTargetPriority=High  SphVelocityTargetValue=[0 0 0]  SphVelocityTargetValueUnits=deg/s  SphVelocityTargetSpecify=off  SphVelocityTargetPriority=High  SphVelocityTargetInFollowerFrame=on
  Base_1_RIGID : Subsystem
  Demux : Demux  Outputs=3
  Ground Contact and Maximum Saturation : Subsystem
  MechanismConfiguration : sm_lib/Utilities/Mechanism Configuration  UniformGravity=Constant  GravityVector=[0 0 -9.8065]  GravityUnits=m/s^2  LinearizationDelta=0.001
  PS Gain : fl_lib/Physical Signals/Functions/PS Gain  gain=-1
  PitchrateConv : nesl_utility/PS-Simulink Converter  PhysicalDomain=network_engine_domain  SubClassName=ps_output  LeftPortType=input  RightPortType=output  PseudoPeriodic=off  Frequencies=[]  Unit=rad/s  AffineConversion=off
  Quaterion : nesl_utility/PS-Simulink Converter  PhysicalDomain=network_engine_domain  SubClassName=ps_output  LeftPortType=input  RightPortType=output  PseudoPeriodic=off  Frequencies=[]  Unit=deg  AffineConversion=off
  Quaternions to Rotation Angles : sharedtransform/Quaternions to Rotation Angles  rotationOrder=XYZ  aMode=aMode
      settings: SourceProductBaseCode=AE
  Rigid Transform : sm_lib/Frames and Transforms/Rigid Transform  TranslationMethod=None  TranslationStandardOffset=0  TranslationLengthUnit=m  TranslationStandardAxis=+Z  TranslationCartesianOffset=[0 0 0]  TranslationROffset=0  TranslationROffsetUnits=m  TranslationZOffset=0  TranslationZOffsetUnits=m  TranslationThetaOffset=0  TranslationThetaOffsetUnits=deg  RotationMethod=None  RotationAngleUnits=deg  RotationStandardAxis=+Z  RotationAngle=0.0  RotationArbitraryAxis=[0 0 1]  FollAlignAxisA=+X  BaseAlignAxisA=+Y  FollAlignAxisB=+Y  BaseAlignAxisB=+Z  RotationSequenceAxes=FollowerAxes  RotationSequence=XYX  RotationSequenceAngles=[0 0 0]  RotationSequenceAnglesUnits=deg  RotationMatrix=[1 0 0; 0 1 0; 0 0 1]
  RollrateConv : nesl_utility/PS-Simulink Converter  PhysicalDomain=network_engine_domain  SubClassName=ps_output  LeftPortType=input  RightPortType=output  PseudoPeriodic=off  Frequencies=[]  Unit=rad/s  AffineConversion=off
  Solver Configuration : nesl_utility/Solver Configuration  PhysicalDomain=network_engine_domain  SubClassName=solver  LeftPortType=input  RightPortType=generic  Tones=[]  Harmonics=[]  SimulateNoise=off  Profile=off  UseLocalSampling=off  EnableSwitchedLinearOptims=on  FrequencyDomain=off  UseCCode=off  RelTol=0.001  AbsTol=1e-06  MinStep=1e-09  ToWorkspace=off  RevertToSquareIcSolve=off  NumHomotopyIterations=100  PhasorMode=off  PhasorModeNumHarmonics=1  DoDC=off  ResidualTolerance=1e-09  UseLocalSolver=off  LocalSolverChoice=NE_BACKWARD_EULER_ADVANCER  LocalSolverSampleTime=0.001  DoFixedCost=off  MaxNonlinIter=3  MaxModeIter=2  LinearAlgebra=Sparse  EquationFormulation=NE_TIME_EF  DelaysMemoryBudget=1024  AutomaticFiltering=on  FilteringTimeConstant=0.001  PartitionStorageMethod=AS_NEEDED  PartitionMemoryBudget=1024  PartitionMethod=FAST
  Transform112 : sm_lib/Frames and Transforms/Rigid Transform  TranslationMethod=Cartesian  TranslationStandardOffset=0  TranslationLengthUnit=m  TranslationStandardAxis=+Z  TranslationCartesianOffset=[-0.0030676637766174002 -0.088943258023244973 0.02756980176226587]  TranslationROffset=0  TranslationROffsetUnits=m  TranslationZOffset=0  TranslationZOffsetUnits=m  TranslationThetaOffset=0  TranslationThetaOffsetUnits=deg  RotationMethod=None  RotationAngleUnits=deg  RotationStandardAxis=+Z  RotationAngle=0.0  RotationArbitraryAxis=[0 0 1]  FollAlignAxisA=+X  BaseAlignAxisA=+Y  FollAlignAxisB=+Y  BaseAlignAxisB=+Z  RotationSequenceAxes=FollowerAxes  RotationSequence=XYX  RotationSequenceAngles=[0 0 0]  RotationSequenceAnglesUnits=deg  RotationMatrix=[1 0 0; 0 1 0; 0 0 1]
  VerticalConv : nesl_utility/PS-Simulink Converter  PhysicalDomain=network_engine_domain  SubClassName=ps_output  LeftPortType=input  RightPortType=output  PseudoPeriodic=off  Frequencies=[]  Unit=m/s  AffineConversion=off
  World : sm_lib/Frames and Transforms/World Frame
  XConv : nesl_utility/PS-Simulink Converter  PhysicalDomain=network_engine_domain  SubClassName=ps_output  LeftPortType=input  RightPortType=output  PseudoPeriodic=off  Frequencies=[]  Unit=m  AffineConversion=off
  YConv : nesl_utility/PS-Simulink Converter  PhysicalDomain=network_engine_domain  SubClassName=ps_output  LeftPortType=input  RightPortType=output  PseudoPeriodic=off  Frequencies=[]  Unit=m  AffineConversion=off
  YawrateConv : nesl_utility/PS-Simulink Converter  PhysicalDomain=network_engine_domain  SubClassName=ps_output  LeftPortType=input  RightPortType=output  PseudoPeriodic=off  Frequencies=[]  Unit=rad/s  AffineConversion=off
  ZConv : nesl_utility/PS-Simulink Converter  PhysicalDomain=network_engine_domain  SubClassName=ps_output  LeftPortType=input  RightPortType=output  PseudoPeriodic=off  Frequencies=[]  Unit=m  AffineConversion=off
  axizlConv : nesl_utility/PS-Simulink Converter  PhysicalDomain=network_engine_domain  SubClassName=ps_output  LeftPortType=input  RightPortType=output  PseudoPeriodic=off  Frequencies=[]  Unit=m/s  AffineConversion=off
  pitch angle fix : Subsystem
  roll angle fix : Subsystem
  sideConv : nesl_utility/PS-Simulink Converter  PhysicalDomain=network_engine_domain  SubClassName=ps_output  LeftPortType=input  RightPortType=output  PseudoPeriodic=off  Frequencies=[]  Unit=m/s  AffineConversion=off
  yaw angle fix : Subsystem
  Tricopter : PMIOPort  Side=Left
  Xlon : Outport
  Ylat : Outport  Port=2
  Zalt : Outport  Port=3
  Vx : Outport  Port=4
  Vy : Outport  Port=5
  Vz : Outport  Port=6
  roll : Outport  Port=7
  pitch : Outport  Port=8
  yaw : Outport  Port=9
  p : Outport  Port=10
  q : Outport  Port=11
  r : Outport  Port=12
  wires:
  YConv/1 -> Ylat/1
  axizlConv/1 -> Vx/1
  sideConv/1 -> Vy/1
  VerticalConv/1 -> Ground Contact and Maximum Saturation/2(V), Vz/1
  RollrateConv/1 -> p/1
  Quaterion/1 -> Quaternions to Rotation Angles/1
  PitchrateConv/1 -> q/1
  YawrateConv/1 -> r/1
  Quaternions to Rotation Angles/1 -> Demux/1
  XConv/1 -> Xlon/1
  ZConv/1 -> Ground Contact and Maximum Saturation/1(Z), Zalt/1
  Demux/1 -> roll angle fix/1(degreeAngle)
  Demux/3 -> yaw angle fix/1(degreeAngle)
  Demux/2 -> pitch angle fix/1(degreeAngle)
  roll angle fix/1(degreeAngleFix) -> roll/1
  pitch angle fix/1(degreeAngleFix) -> pitch/1
  yaw angle fix/1(degreeAngleFix) -> yaw/1
  connections:
  Base_1_RIGID/LConn1 -- Transform112/RConn1
  Transform112/LConn1 -- Rigid Transform/LConn1 -- Solver Configuration/RConn1 -- MechanismConfiguration/RConn1 -- World/RConn1
  6-DOF Joint/RConn1 -- Tricopter/RConn1
  XConv/LConn1 -- 6-DOF Joint/RConn2
  YConv/LConn1 -- 6-DOF Joint/RConn4
  PS Gain/LConn1 -- 6-DOF Joint/RConn6
  axizlConv/LConn1 -- 6-DOF Joint/RConn3
  sideConv/LConn1 -- 6-DOF Joint/RConn5
  VerticalConv/LConn1 -- 6-DOF Joint/RConn7
  RollrateConv/LConn1 -- 6-DOF Joint/RConn9
  6-DOF Joint/RConn8 -- Quaterion/LConn1
  YawrateConv/LConn1 -- 6-DOF Joint/RConn11
  6-DOF Joint/RConn10 -- PitchrateConv/LConn1
  Ground Contact and Maximum Saturation/RConn1 -- 6-DOF Joint/LConn2
  ZConv/LConn1 -- PS Gain/RConn1
  Rigid Transform/RConn1 -- 6-DOF Joint/LConn1

== system TriTiltPro_V3/ASingle-Tilt Tricopter 3D Model/Tricopter ==
  Ul : Inport
  Ur : Inport  Port=2
  Ut : Inport  Port=3
  Uti : Inport  Port=4
  Frame : Subsystem
  Left Rotor : Subsystem
  Right Rotor : Subsystem
  Tail Rotor : Subsystem
  WorldBase : PMIOPort  Side=Right
  wires:
  Ur/1 -> Right Rotor/1(Ur)
  Ul/1 -> Left Rotor/1(Ul)
  Ut/1 -> Tail Rotor/1(Ut)
  Uti/1 -> Tail Rotor/2(Uti)
  connections:
  Frame/LConn1 -- Left Rotor/RConn1 -- Right Rotor/RConn1 -- WorldBase/RConn1 -- Tail Rotor/RConn1

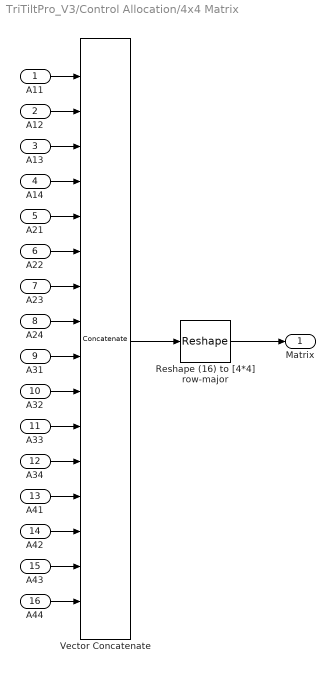
== system TriTiltPro_V3/Control Allocation/4x4 Matrix ==
  A11 : Inport
  A12 : Inport  Port=2
  A13 : Inport  Port=3
  A14 : Inport  Port=4
  A21 : Inport  Port=5
  A22 : Inport  Port=6
  A23 : Inport  Port=7
  A24 : Inport  Port=8
  A31 : Inport  Port=9
  A32 : Inport  Port=10
  A33 : Inport  Port=11
  A34 : Inport  Port=12
  A41 : Inport  Port=13
  A42 : Inport  Port=14
  A43 : Inport  Port=15
  A44 : Inport  Port=16
  Reshape (16) to [4*4] row-major : Reshape  OutputDimensionality=Customize  OutputDimensions=[4,4]
  Vector Concatenate : Concatenate  NumInputs=16
  Matrix : Outport
  wires:
  Vector Concatenate/1 -> Reshape (16) to [4*4] row-major/1
  A11/1 -> Vector Concatenate/1
  A12/1 -> Vector Concatenate/2
  A13/1 -> Vector Concatenate/3
  A14/1 -> Vector Concatenate/4
  A21/1 -> Vector Concatenate/5
  A22/1 -> Vector Concatenate/6
  A23/1 -> Vector Concatenate/7
  A24/1 -> Vector Concatenate/8
  A33/1 -> Vector Concatenate/11
  A31/1 -> Vector Concatenate/9
  A32/1 -> Vector Concatenate/10
  A34/1 -> Vector Concatenate/12
  A41/1 -> Vector Concatenate/13
  A42/1 -> Vector Concatenate/14
  A43/1 -> Vector Concatenate/15
  A44/1 -> Vector Concatenate/16
  Reshape (16) to [4*4] row-major/1 -> Matrix/1

== system TriTiltPro_V3/Control Allocation/Invert 4x4 Matrix ==
  MatrixIn : Inport
  Assertion1 : Assertion  AssertionFailFcn="disp('Matrix is singular.  No matrix inverse.')"
  Determinant of a 4x4 Matrix : Subsystem
      mask Display: disp('det(A)(4x4)');
  Product : Product  Inputs=/  Multiplication=Matrix(*)
  InvMatrix : Outport
  wires:
  Determinant of a 4x4 Matrix/1(Det(Matrix)) -> Assertion1/1
  MatrixIn/1 -> Product/1, Determinant of a 4x4 Matrix/1(MatrixIn)
  Product/1 -> InvMatrix/1

== system TriTiltPro_V3/Position Control/Outer Error Ports ==
  Reference Inputs : Inport
  Outputs : Inport  Port=2
  Demux : Demux  Outputs=3
  Demux1 : Demux  Outputs=6
  Mux : Mux  Inputs=3
  Mux2 : Mux  Inputs=1
  Sum : Sum  Inputs=|+-
  Sum1 : Sum  Inputs=|+-
  Sum2 : Sum  Inputs=|+-
  Terminator : Terminator
  Terminator1 : Terminator
  Terminator2 : Terminator
  Errors : Outport
  wires:
  Outputs/1 -> Demux1/1
  Reference Inputs/1 -> Demux/1
  Demux/2 -> Sum1/1  "longitude cmd"
  Demux/3 -> Sum2/1  "Altitude cmd"
  Demux1/1 -> Sum/2  "X"
  Demux1/2 -> Sum1/2  "Y"
  Demux1/3 -> Sum2/2  "Altitude"
  Sum2/1 -> Mux/3  "errAltitude"
  Sum1/1 -> Mux/2  "errY"
  Sum/1 -> Mux/1  "errX"
  Demux/1 -> Sum/1  "latitude cmd"
  Mux/1 -> Mux2/1  "errors"
  Mux2/1 -> Errors/1
  Demux1/4 -> Terminator/1
  Demux1/5 -> Terminator1/1
  Demux1/6 -> Terminator2/1
